simulink model "hexActuator"  (R2024a)
settings: configuration reference "standardSILConfiguraitonParams" (kept outside this file)
settings Model: Creator=jerem  LastModifiedBy=jerem
settings ConfigSetRef: SourceName=standardSILConfiguraitonParams  SourceLocation=Base Workspace

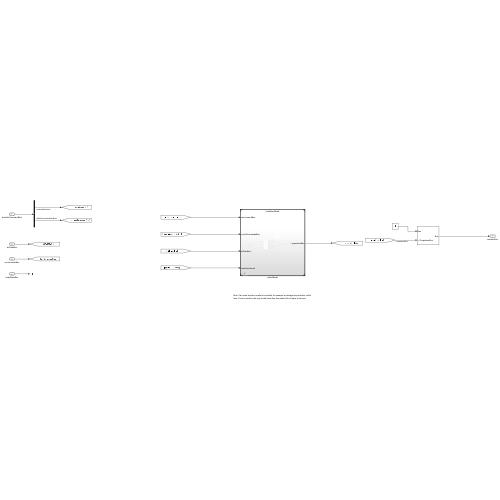
[thumbnail: Simulink's stored preview of the top-level diagram]
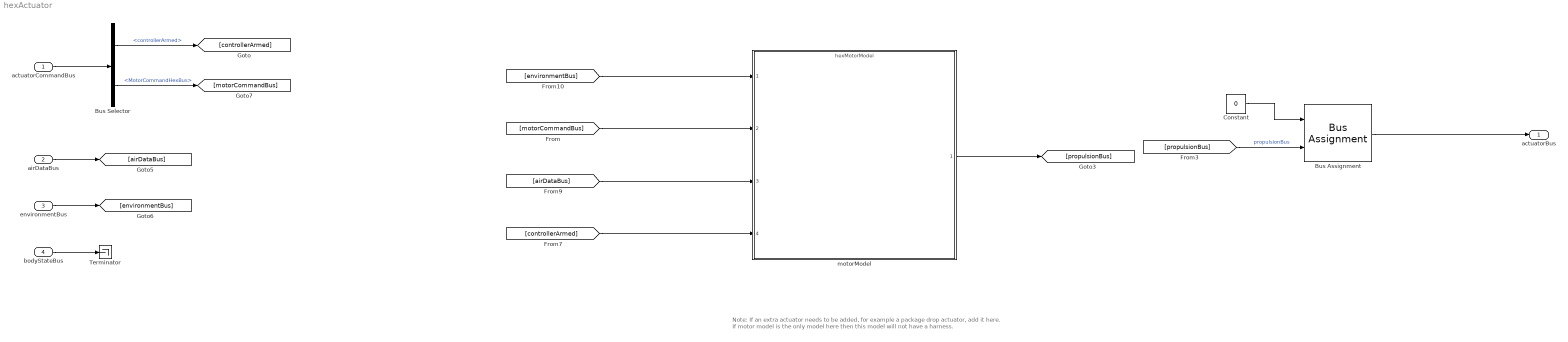
== system hexActuator ==
  note: Note: If an extra actuator needs to be added, for example a package drop actuator, add it here. If motor model is the only model here then this model will not have a harness.
  actuatorCommandBus : Inport  OutDataTypeStr=Bus: ActuatorCommandBus
  airDataBus : Inport  Port=2  OutDataTypeStr=Bus: AirDataBus
  environmentBus : Inport  Port=3  OutDataTypeStr=Bus: EnvironmentBus
  bodyStateBus : Inport  Port=4  OutDataTypeStr=Bus: BodyStateBus
  Bus Assignment : BusAssignment  AssignedSignals=PropulsionBus
  Bus Selector : BusSelector  OutputSignals=controllerArmed,ServosCommandBus.MotorCommandHexBus
  Constant : Constant  Value=0  OutDataTypeStr=Bus: ActuatorBus
  Terminator : Terminator
  motorModel : ModelReference  ModelNameDialog=hexMotorModel.slx  SimulationMode=Normal  ModelReferenceVersion=1.180
  actuatorBus : Outport  OutDataTypeStr=Bus: ActuatorBus
  wires:
  actuatorCommandBus/1 -> Bus Selector/1
  Bus Selector/2 -> [motorCommandBus]  "<MotorCommandHexBus>"
  environmentBus/1 -> [environmentBus]
  bodyStateBus/1 -> Terminator/1
  airDataBus/1 -> [airDataBus]
  Bus Selector/1 -> [controllerArmed]  "<controllerArmed>"
  Bus Assignment/1 -> actuatorBus/1
  motorModel/1 -> [propulsionBus]
  [propulsionBus] -> Bus Assignment/2  "propulsionBus"
  Constant/1 -> Bus Assignment/1
  [controllerArmed] -> motorModel/4
  [motorCommandBus] -> motorModel/2
  [environmentBus] -> motorModel/1
  [airDataBus] -> motorModel/3
